simulink model "MedianFilter_cam_front"  (R2018b)
settings: Solver=FixedStepAuto  StartTime=0.0  StopTime=inf  FixedStep=0.05  RelTol=1e-3
model workspace (MAT data in the model file):
  SL_ROS_VariableLengthArrays_MaxSizes.CommonInfo.ArrayTruncateAction = 'EmitWarning'
  SL_ROS_VariableLengthArrays_MaxSizes.MsgTypeMap = containers.Map
  SL_ROS_VariableLengthArrays_MaxSizes.MsgTypeMap.serialization.keys = {'sensor_msgs/Image'}
  SL_ROS_VariableLengthArrays_MaxSizes.MsgTypeMap.serialization.values{1}(1).PropertyName = 'Data'
  SL_ROS_VariableLengthArrays_MaxSizes.MsgTypeMap.serialization.values{1}(1).DataType = 'uint8'
  SL_ROS_VariableLengthArrays_MaxSizes.MsgTypeMap.serialization.values{1}(1).MaxLength = 1036800
  SL_ROS_VariableLengthArrays_MaxSizes.MsgTypeMap.serialization.values{1}(2).PropertyName = 'Encoding'
  SL_ROS_VariableLengthArrays_MaxSizes.MsgTypeMap.serialization.values{1}(2).DataType = 'uint8'
  SL_ROS_VariableLengthArrays_MaxSizes.MsgTypeMap.serialization.values{1}(2).MaxLength = 1036800
  SL_ROS_VariableLengthArrays_MaxSizes.MsgTypeMap.serialization.uniformity = 0
  SL_ROS_VariableLengthArrays_MaxSizes.MsgTypeMap.serialization.keyType = 'char'
  SL_ROS_VariableLengthArrays_MaxSizes.MsgTypeMap.serialization.valueType = 'any'
undefined symbols (not defined in the file or in its folder): Data, Data_SL_Info, Encoding, Encoding_SL_Info, Header, Height, IsBigendian, Step, Width
libraries: robotlib x3, svdutilitieslib x2, visionanalysis x1
settings Model: Creator=HannesDittmann  LastModifiedBy=alf
settings OptimizationCC: EnhancedBackFolding=on  PassReuseOutputArgsAs=Individual arguments  MaxStackSize=64  OptimizeBlockOrder=speed  DifferentSizesBufferReuse=on  OptimizationCustomize=off
settings DebuggingCC: ParameterTunabilityLossMsg=error  UnderSpecifiedDimensionMsg=warning
settings HardwareCC: ProdBitPerPointer=32  ProdBitPerSizeT=32  ProdBitPerPtrDiffT=32  ProdLargestAtomicFloat=None  ProdIntDivRoundTo=Undefined  ProdEndianess=Unspecified  ProdWordSize=32  ProdHWDeviceType=Generic->Unspecified (assume 32-bit Generic)
settings SFSimCC: MATLABDynamicMemAlloc=off
settings RTWCC: SystemTargetFile=ert.tlc  HardwareBoard=Robot Operating System (ROS)  TLCOptions="-aInlineSetEventsForThisBaseRateFcn=TLC_FALSE -aSuppressMultiTaskScheduler=TLC_FALSE  -aRateBasedStepFcn=0"  TemplateMakefile=ert_default_tmf  GenerateReport=on  Toolchain=Catkin  IncludeHyperlinkInReport=on  LaunchReport=on  TargetLang=C++  GenerateTraceInfo=on  GenerateTraceReport=on  GenerateTraceReportSl=on  GenerateTraceReportSf=on  GenerateTraceReportEml=on
settings CodeAppCC: ForceParamTrailComments=on  IgnoreCustomStorageClasses=off  OperatorAnnotations=on  SimulinkDataObjDesc=on  SFDataObjDesc=on  InsertBlockDesc=on
settings ERTTargetCC: SupportVariableSizeSignals=on

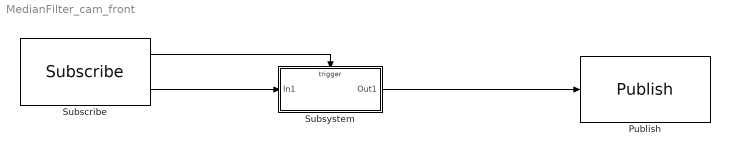
== system MedianFilter_cam_front ==
  Publish : robotlib/Publish  topicSource=Specify your own  topic=/kinect2/qhd/depth_image_filtered  messageType=sensor_msgs/Image  messageQueueLength=1
      settings: SourceProductBaseCode=RO
  Subscribe : robotlib/Subscribe  topicSource=Specify your own  topic=/kinect2/qhd/image_depth_rect  messageType=sensor_msgs/Image  sampleTime=0.1  messageQueueLength=1
      settings: SourceProductBaseCode=RO
  Subsystem : Subsystem
  wires:
  Subscribe/2 -> Subsystem/1(In1)
  Subsystem/1(Out1) -> Publish/1
  Subscribe/1 -> Subsystem/Trigger

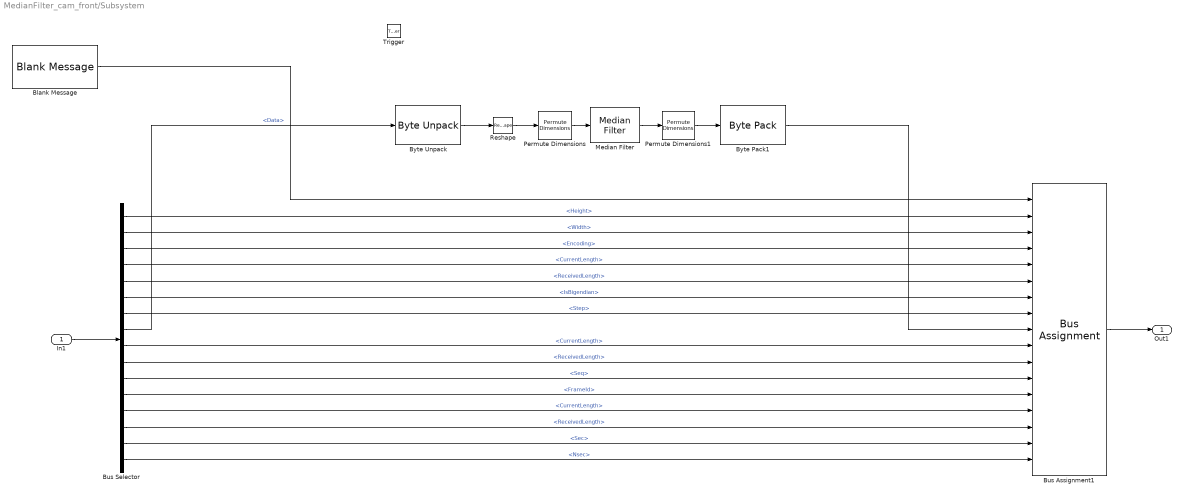
== system MedianFilter_cam_front/Subsystem ==
  In1 : Inport
  Trigger : TriggerPort  VariantControl=Variant  PortDimensions=1
  Blank Message : robotlib/Blank Message  messageClass=Message  entityType=sensor_msgs/Image  messageType=sensor_msgs/Image  SampleTime=-1
      settings: SourceProductBaseCode=RO
  Bus Assignment1 : BusAssignment  AssignedSignals=Height,Width,Encoding,Encoding_SL_Info.CurrentLength,Encoding_SL_Info.ReceivedLength,IsBigendian,Step,Data,Data_SL_Info.CurrentLength,Data_SL_Info.ReceivedLength,Header.Seq,Header.FrameId,Header.FrameId_SL_Info.CurrentLength,Header.FrameId_SL_Info.ReceivedLength,Header.Stamp.Sec,Header.Stamp.Nsec
  Bus Selector : BusSelector  OutputSignals=Height,Width,Encoding,Encoding_SL_Info.CurrentLength,Encoding_SL_Info.ReceivedLength,IsBigendian,Step,Data,Data_SL_Info.CurrentLength,Data_SL_Info.ReceivedLength,Header.Seq,Header.FrameId,Header.FrameId_SL_Info.CurrentLength,Header.FrameId_SL_Info.ReceivedLength,Header.Stamp.Sec,Header.Stamp.Nsec
  Byte Pack1 : svdutilitieslib/Byte Pack  maskPackedDataType=uint8  datatypes={'uint16'}  byteAlign=1  blockPlatform=arduinoert
      settings: SourceProductName=Simulink Support Package for Arduino Hardware  SourceProductBaseCode=ARDUINO
  Byte Unpack : svdutilitieslib/Byte Unpack  dimensions={[518400]}  datatypes={'uint16'}  byteAlign=1  blockPlatform=arduinoert
      settings: SourceProductName=Simulink Support Package for Arduino Hardware  SourceProductBaseCode=ARDUINO
  Median Filter : visionanalysis/Median Filter  nghbood=[5]  outSize=Same as input port I  padType=Symmetric  padSrc=Specify via dialog  padVal=0  roundingMode=Floor  overflowMode=off
      settings: SourceProductName=Computer Vision System Toolbox  SourceProductBaseCode=VP
  Permute Dimensions : PermuteDimensions
  Permute Dimensions1 : PermuteDimensions
  Reshape : Reshape  OutputDimensionality=Customize  OutputDimensions=[960,540]
  Out1 : Outport
  wires:
  Bus Selector/9 -> Bus Assignment1/10  "<CurrentLength>"
  Byte Unpack/1 -> Reshape/1
  Bus Selector/3 -> Bus Assignment1/4  "<Encoding>"
  Bus Selector/15 -> Bus Assignment1/16  "<Sec>"
  Bus Selector/6 -> Bus Assignment1/7  "<IsBigendian>"
  Permute Dimensions/1 -> Median Filter/1
  Bus Selector/12 -> Bus Assignment1/13  "<FrameId>"
  Bus Selector/10 -> Bus Assignment1/11  "<ReceivedLength>"
  Bus Selector/7 -> Bus Assignment1/8  "<Step>"
  Reshape/1 -> Permute Dimensions/1
  Bus Selector/13 -> Bus Assignment1/14  "<CurrentLength>"
  Median Filter/1 -> Permute Dimensions1/1
  Bus Selector/5 -> Bus Assignment1/6  "<ReceivedLength>"
  Bus Selector/14 -> Bus Assignment1/15  "<ReceivedLength>"
  Bus Selector/8 -> Byte Unpack/1  "<Data>"
  Bus Selector/16 -> Bus Assignment1/17  "<Nsec>"
  Bus Selector/4 -> Bus Assignment1/5  "<CurrentLength>"
  Bus Selector/2 -> Bus Assignment1/3  "<Width>"
  Bus Selector/11 -> Bus Assignment1/12  "<Seq>"
  Byte Pack1/1 -> Bus Assignment1/9
  Permute Dimensions1/1 -> Byte Pack1/1
  Bus Selector/1 -> Bus Assignment1/2  "<Height>"
  Bus Assignment1/1 -> Out1/1
  In1/1 -> Bus Selector/1
  Blank Message/1 -> Bus Assignment1/1
